simulink library "gbt_library"  (Simulink 7.4)
settings: Solver=ode45  StartTime=0.0  StopTime=10.0  RelTol=1e-3
libraries: xbsIndex_r4 x1525, casper_library_flow_control x20, casper_library_misc x15, xps_library x1
(part 4 of 14)

== system gbt_library/Parallel_CIC_filter_stage/comb_2 ==
  sync_in : Inport
  in1 : Inport  Port=2
  in2 : Inport  Port=3
  Delay2 : xbsIndex_r4/Delay  en=off  latency=1  dbl_ovrd=off  reg_retiming=off  block_type=delay
      settings: block_version=11.4
  sub_blk1 : xbsIndex_r4/AddSub  mode=Subtraction  use_carryin=off  use_carryout=off  en=off  latency=1  precision=User Defined  arith_type="Signed  (2's comp)"  n_bits=13  bin_pt=7  quantization=Truncate  overflow=Wrap  dbl_ovrd=off  use_behavioral_HDL=on  hw_selection=Fabric  pipelined=off  block_type=addsub
  sub_blk2 : xbsIndex_r4/AddSub  mode=Subtraction  use_carryin=off  use_carryout=off  en=off  latency=1  precision=User Defined  arith_type="Signed  (2's comp)"  n_bits=13  bin_pt=7  quantization=Truncate  overflow=Wrap  dbl_ovrd=off  use_behavioral_HDL=on  hw_selection=Fabric  pipelined=off  block_type=addsub
  sync_delay : xbsIndex_r4/Delay  en=off  latency=1  dbl_ovrd=off  reg_retiming=off  block_type=delay
      settings: block_version=11.4
  sync_out : Outport
  out1 : Outport  Port=2
  out2 : Outport  Port=3
  wires:
  in2/1 -> sub_blk2/1, Delay2/1
  in1/1 -> sub_blk2/2, sub_blk1/1
  sync_delay/1 -> sync_out/1
  sync_in/1 -> sync_delay/1
  sub_blk2/1 -> out2/1
  sub_blk1/1 -> out1/1
  Delay2/1 -> sub_blk1/2  "d_in2"

== system gbt_library/Parallel_CIC_filter_stage/comb_3 ==
  sync_in : Inport
  in1 : Inport  Port=2
  in2 : Inport  Port=3
  Delay2 : xbsIndex_r4/Delay  en=off  latency=1  dbl_ovrd=off  reg_retiming=off  block_type=delay
      settings: block_version=11.4
  sub_blk1 : xbsIndex_r4/AddSub  mode=Subtraction  use_carryin=off  use_carryout=off  en=off  latency=1  precision=User Defined  arith_type="Signed  (2's comp)"  n_bits=13  bin_pt=7  quantization=Truncate  overflow=Wrap  dbl_ovrd=off  use_behavioral_HDL=on  hw_selection=Fabric  pipelined=off  block_type=addsub
  sub_blk2 : xbsIndex_r4/AddSub  mode=Subtraction  use_carryin=off  use_carryout=off  en=off  latency=1  precision=User Defined  arith_type="Signed  (2's comp)"  n_bits=13  bin_pt=7  quantization=Truncate  overflow=Wrap  dbl_ovrd=off  use_behavioral_HDL=on  hw_selection=Fabric  pipelined=off  block_type=addsub
  sync_delay : xbsIndex_r4/Delay  en=off  latency=1  dbl_ovrd=off  reg_retiming=off  block_type=delay
      settings: block_version=11.4
  sync_out : Outport
  out1 : Outport  Port=2
  out2 : Outport  Port=3
  wires:
  in2/1 -> sub_blk2/1, Delay2/1
  in1/1 -> sub_blk2/2, sub_blk1/1
  sync_delay/1 -> sync_out/1
  sync_in/1 -> sync_delay/1
  sub_blk2/1 -> out2/1
  sub_blk1/1 -> out1/1
  Delay2/1 -> sub_blk1/2  "d_in2"

== system gbt_library/Parallel_CIC_filter_stage/downsample_3 ==
  sync_in : Inport
  In1 : Inport  Port=2
  In2 : Inport  Port=3
  Down_sample1 : xbsIndex_r4/Down Sample  sample_ratio=3  sample_phase="Last Value of Frame  (most efficient)"  en=off  latency=1  dbl_ovrd=off  block_type=dsamp
      settings: block_version=11.4
  Down_sample2 : xbsIndex_r4/Down Sample  sample_ratio=3  sample_phase="Last Value of Frame  (most efficient)"  en=off  latency=1  dbl_ovrd=off  block_type=dsamp
      settings: block_version=11.4
  delay1 : xbsIndex_r4/Delay  en=off  latency=1  dbl_ovrd=off  reg_retiming=off  block_type=delay
      settings: block_version=11.4
  delay2 : xbsIndex_r4/Delay  en=off  latency=0  dbl_ovrd=off  reg_retiming=off  block_type=delay
      settings: block_version=11.4
  sync_delay : xbsIndex_r4/Delay  en=off  latency=1  dbl_ovrd=off  reg_retiming=off  block_type=delay
      settings: block_version=11.4
  sync_out : Outport
  Out1 : Outport  Port=2
  Out2 : Outport  Port=3
  wires:
  sync_delay/1 -> sync_out/1
  sync_in/1 -> sync_delay/1
  Down_sample2/1 -> Out2/1
  delay2/1 -> Down_sample2/1  "dO2"
  In2/1 -> delay2/1
  Down_sample1/1 -> Out1/1
  delay1/1 -> Down_sample1/1  "dO1"
  In1/1 -> delay1/1

== system gbt_library/Parallel_CIC_filter_stage/int_1 ==
  in1 : Inport
  in2 : Inport  Port=2
  sync : Inport  Port=3
  Accumulator1 : xbsIndex_r4/Accumulator  operation=Add  n_bits=13  overflow=Wrap  scale=1  rst=off  hasbypass=off  en=off  dbl_ovrd=off  use_behavioral_HDL=on  implementation=Fabric  block_type=accum
      settings: block_version=11.4
  Accumulator2 : xbsIndex_r4/Accumulator  operation=Add  n_bits=13  overflow=Wrap  scale=1  rst=off  hasbypass=off  en=off  dbl_ovrd=off  use_behavioral_HDL=on  implementation=Fabric  block_type=accum
      settings: block_version=11.4
  Delay2 : xbsIndex_r4/Delay  en=off  latency=1  dbl_ovrd=off  reg_retiming=off  block_type=delay
      settings: block_version=11.4
  adder_tree1 : Subsystem
  adder_tree2 : Subsystem
  out1 : Outport
  out2 : Outport  Port=2
  wires:
  Accumulator2/1 -> adder_tree2/3(din_2), Delay2/1  "Im2"
  sync/1 -> adder_tree2/1(sync), adder_tree1/1(sync)
  Accumulator1/1 -> adder_tree2/2(din_1), adder_tree1/2(din_1)  "Im1"
  adder_tree2/2(dout) -> out2/1
  adder_tree1/2(dout) -> out1/1
  Delay2/1 -> adder_tree1/3(din_2)  "dIm2"
  in2/1 -> Accumulator2/1
  in1/1 -> Accumulator1/1

== system gbt_library/Parallel_CIC_filter_stage/int_2 ==
  in1 : Inport
  in2 : Inport  Port=2
  sync : Inport  Port=3
  Accumulator1 : xbsIndex_r4/Accumulator  operation=Add  n_bits=13  overflow=Wrap  scale=1  rst=off  hasbypass=off  en=off  dbl_ovrd=off  use_behavioral_HDL=on  implementation=Fabric  block_type=accum
      settings: block_version=11.4
  Accumulator2 : xbsIndex_r4/Accumulator  operation=Add  n_bits=13  overflow=Wrap  scale=1  rst=off  hasbypass=off  en=off  dbl_ovrd=off  use_behavioral_HDL=on  implementation=Fabric  block_type=accum
      settings: block_version=11.4
  Delay2 : xbsIndex_r4/Delay  en=off  latency=1  dbl_ovrd=off  reg_retiming=off  block_type=delay
      settings: block_version=11.4
  adder_tree1 : Subsystem
  adder_tree2 : Subsystem
  out1 : Outport
  out2 : Outport  Port=2
  wires:
  Accumulator2/1 -> adder_tree2/3(din_2), Delay2/1  "Im2"
  sync/1 -> adder_tree2/1(sync), adder_tree1/1(sync)
  Accumulator1/1 -> adder_tree2/2(din_1), adder_tree1/2(din_1)  "Im1"
  adder_tree2/2(dout) -> out2/1
  adder_tree1/2(dout) -> out1/1
  Delay2/1 -> adder_tree1/3(din_2)  "dIm2"
  in2/1 -> Accumulator2/1
  in1/1 -> Accumulator1/1

== system gbt_library/Parallel_CIC_filter_stage/int_3 ==
  in1 : Inport
  in2 : Inport  Port=2
  sync : Inport  Port=3
  Accumulator1 : xbsIndex_r4/Accumulator  operation=Add  n_bits=13  overflow=Wrap  scale=1  rst=off  hasbypass=off  en=off  dbl_ovrd=off  use_behavioral_HDL=on  implementation=Fabric  block_type=accum
      settings: block_version=11.4
  Accumulator2 : xbsIndex_r4/Accumulator  operation=Add  n_bits=13  overflow=Wrap  scale=1  rst=off  hasbypass=off  en=off  dbl_ovrd=off  use_behavioral_HDL=on  implementation=Fabric  block_type=accum
      settings: block_version=11.4
  Delay2 : xbsIndex_r4/Delay  en=off  latency=1  dbl_ovrd=off  reg_retiming=off  block_type=delay
      settings: block_version=11.4
  adder_tree1 : Subsystem
  adder_tree2 : Subsystem
  out1 : Outport
  out2 : Outport  Port=2
  wires:
  Accumulator2/1 -> adder_tree2/3(din_2), Delay2/1  "Im2"
  sync/1 -> adder_tree2/1(sync), adder_tree1/1(sync)
  Accumulator1/1 -> adder_tree2/2(din_1), adder_tree1/2(din_1)  "Im1"
  adder_tree2/2(dout) -> out2/1
  adder_tree1/2(dout) -> out1/1
  Delay2/1 -> adder_tree1/3(din_2)  "dIm2"
  in2/1 -> Accumulator2/1
  in1/1 -> Accumulator1/1

== system gbt_library/Spacketizer/parallel_to_serial_converter ==
  pin : Inport
  ld : Inport  Port=2
  shift : Inport  Port=3
  Logical : xbsIndex_r4/Logical  logical_function=OR  inputs=2  en=off  latency=0  precision=Full  arith_type=Unsigned  n_bits=16  bin_pt=0  align_bp=on  dbl_ovrd=off  block_type=logical
  filler : xbsIndex_r4/Constant  arith_type=Unsigned  const=0  n_bits=sout_width  bin_pt=0  explicit_period=on  period=1  equ=P=C  opselect=C  inp2=PCIN>>17  opr=+  inp1=P  carry=CIN  dbl_ovrd=off  block_type=constant
  shifter_unit1 : casper_library_flow_control/shifter_unit  SystemSampleTime=-1  data_width=64  pin_offset=0
  shifter_unit2 : casper_library_flow_control/shifter_unit  SystemSampleTime=-1  data_width=64  pin_offset=64
  shifter_unit3 : casper_library_flow_control/shifter_unit  SystemSampleTime=-1  data_width=64  pin_offset=128
  shifter_unit4 : casper_library_flow_control/shifter_unit  SystemSampleTime=-1  data_width=64  pin_offset=192
  sout : Outport  OutDataType=sfix(16)  OutScaling=2^0
  wires:
  shifter_unit4/1 -> sout/1
  shifter_unit3/1 -> shifter_unit4/2
  shifter_unit2/1 -> shifter_unit3/2
  shifter_unit1/1 -> shifter_unit2/2
  Logical/1 -> shifter_unit4/4, shifter_unit3/4, shifter_unit2/4, shifter_unit1/4
  pin/1 -> shifter_unit4/3, shifter_unit3/3, shifter_unit2/3, shifter_unit1/3
  filler/1 -> shifter_unit1/2
  shift/1 -> Logical/2
  ld/1 -> shifter_unit4/1, shifter_unit3/1, shifter_unit2/1, shifter_unit1/1, Logical/1

== system gbt_library/halfband/adder_tree ==
  sync : Inport
  din1 : Inport  Port=2
  din2 : Inport  Port=3
  din3 : Inport  Port=4
  din4 : Inport  Port=5
  addr1 : xbsIndex_r4/AddSub  mode=Addition  use_carryin=off  use_carryout=off  en=off  latency=1  precision=Full  arith_type=Unsigned  n_bits=16  bin_pt=14  quantization=Truncate  overflow=Wrap  dbl_ovrd=off  use_behavioral_HDL=off  hw_selection=Fabric  pipelined=on  use_rpm=on  block_type=addsub
  addr2 : xbsIndex_r4/AddSub  mode=Addition  use_carryin=off  use_carryout=off  en=off  latency=1  precision=Full  arith_type=Unsigned  n_bits=16  bin_pt=14  quantization=Truncate  overflow=Wrap  dbl_ovrd=off  use_behavioral_HDL=off  hw_selection=Fabric  pipelined=on  use_rpm=on  block_type=addsub
  addr3 : xbsIndex_r4/AddSub  mode=Addition  use_carryin=off  use_carryout=off  en=off  latency=1  precision=Full  arith_type=Unsigned  n_bits=16  bin_pt=14  quantization=Truncate  overflow=Wrap  dbl_ovrd=off  use_behavioral_HDL=off  hw_selection=Fabric  pipelined=on  use_rpm=on  block_type=addsub
  sync_delay : xbsIndex_r4/Delay  en=off  latency=2  dbl_ovrd=off  reg_retiming=on  block_type=delay
      settings: block_version=11.4
  sync_out : Outport
  dout : Outport  Port=2
  wires:
  addr3/1 -> dout/1  "adder_outs2_1"
  addr2/1 -> addr3/2  "adder_outs1_2"
  addr1/1 -> addr3/1  "adder_outs1_1"
  din4/1 -> addr2/2
  din3/1 -> addr2/1
  din2/1 -> addr1/2
  din1/1 -> addr1/1
  sync_delay/1 -> sync_out/1
  sync/1 -> sync_delay/1

== system gbt_library/halfband/adder_tree1 ==
  sync : Inport
  din1 : Inport  Port=2
  din2 : Inport  Port=3
  din3 : Inport  Port=4
  din4 : Inport  Port=5
  addr1 : xbsIndex_r4/AddSub  mode=Addition  use_carryin=off  use_carryout=off  en=off  latency=1  precision=Full  arith_type=Unsigned  n_bits=16  bin_pt=14  quantization=Truncate  overflow=Wrap  dbl_ovrd=off  use_behavioral_HDL=off  hw_selection=Fabric  pipelined=on  use_rpm=on  block_type=addsub
  addr2 : xbsIndex_r4/AddSub  mode=Addition  use_carryin=off  use_carryout=off  en=off  latency=1  precision=Full  arith_type=Unsigned  n_bits=16  bin_pt=14  quantization=Truncate  overflow=Wrap  dbl_ovrd=off  use_behavioral_HDL=off  hw_selection=Fabric  pipelined=on  use_rpm=on  block_type=addsub
  addr3 : xbsIndex_r4/AddSub  mode=Addition  use_carryin=off  use_carryout=off  en=off  latency=1  precision=Full  arith_type=Unsigned  n_bits=16  bin_pt=14  quantization=Truncate  overflow=Wrap  dbl_ovrd=off  use_behavioral_HDL=off  hw_selection=Fabric  pipelined=on  use_rpm=on  block_type=addsub
  sync_delay : xbsIndex_r4/Delay  en=off  latency=2  dbl_ovrd=off  reg_retiming=on  block_type=delay
      settings: block_version=11.4
  sync_out : Outport
  dout : Outport  Port=2
  wires:
  addr3/1 -> dout/1  "adder_outs2_1"
  addr2/1 -> addr3/2  "adder_outs1_2"
  addr1/1 -> addr3/1  "adder_outs1_1"
  din4/1 -> addr2/2
  din3/1 -> addr2/1
  din2/1 -> addr1/2
  din1/1 -> addr1/1
  sync_delay/1 -> sync_out/1
  sync/1 -> sync_delay/1

== system gbt_library/halfband/adder_tree3 ==
  sync : Inport
  din1 : Inport  Port=2
  din2 : Inport  Port=3
  din3 : Inport  Port=4
  din4 : Inport  Port=5
  addr1 : xbsIndex_r4/AddSub  mode=Addition  use_carryin=off  use_carryout=off  en=off  latency=1  precision=Full  arith_type=Unsigned  n_bits=16  bin_pt=14  quantization=Truncate  overflow=Wrap  dbl_ovrd=off  use_behavioral_HDL=off  hw_selection=Fabric  pipelined=on  use_rpm=on  block_type=addsub
  addr2 : xbsIndex_r4/AddSub  mode=Addition  use_carryin=off  use_carryout=off  en=off  latency=1  precision=Full  arith_type=Unsigned  n_bits=16  bin_pt=14  quantization=Truncate  overflow=Wrap  dbl_ovrd=off  use_behavioral_HDL=off  hw_selection=Fabric  pipelined=on  use_rpm=on  block_type=addsub
  addr3 : xbsIndex_r4/AddSub  mode=Addition  use_carryin=off  use_carryout=off  en=off  latency=1  precision=Full  arith_type=Unsigned  n_bits=16  bin_pt=14  quantization=Truncate  overflow=Wrap  dbl_ovrd=off  use_behavioral_HDL=off  hw_selection=Fabric  pipelined=on  use_rpm=on  block_type=addsub
  sync_delay : xbsIndex_r4/Delay  en=off  latency=2  dbl_ovrd=off  reg_retiming=on  block_type=delay
      settings: block_version=11.4
  sync_out : Outport
  dout : Outport  Port=2
  wires:
  addr3/1 -> dout/1  "adder_outs2_1"
  addr2/1 -> addr3/2  "adder_outs1_2"
  addr1/1 -> addr3/1  "adder_outs1_1"
  din4/1 -> addr2/2
  din3/1 -> addr2/1
  din2/1 -> addr1/2
  din1/1 -> addr1/1
  sync_delay/1 -> sync_out/1
  sync/1 -> sync_delay/1

== system gbt_library/halfband/adder_tree4 ==
  sync : Inport
  din1 : Inport  Port=2
  din2 : Inport  Port=3
  din3 : Inport  Port=4
  din4 : Inport  Port=5
  addr1 : xbsIndex_r4/AddSub  mode=Addition  use_carryin=off  use_carryout=off  en=off  latency=1  precision=Full  arith_type=Unsigned  n_bits=16  bin_pt=14  quantization=Truncate  overflow=Wrap  dbl_ovrd=off  use_behavioral_HDL=off  hw_selection=Fabric  pipelined=on  use_rpm=on  block_type=addsub
  addr2 : xbsIndex_r4/AddSub  mode=Addition  use_carryin=off  use_carryout=off  en=off  latency=1  precision=Full  arith_type=Unsigned  n_bits=16  bin_pt=14  quantization=Truncate  overflow=Wrap  dbl_ovrd=off  use_behavioral_HDL=off  hw_selection=Fabric  pipelined=on  use_rpm=on  block_type=addsub
  addr3 : xbsIndex_r4/AddSub  mode=Addition  use_carryin=off  use_carryout=off  en=off  latency=1  precision=Full  arith_type=Unsigned  n_bits=16  bin_pt=14  quantization=Truncate  overflow=Wrap  dbl_ovrd=off  use_behavioral_HDL=off  hw_selection=Fabric  pipelined=on  use_rpm=on  block_type=addsub
  sync_delay : xbsIndex_r4/Delay  en=off  latency=2  dbl_ovrd=off  reg_retiming=on  block_type=delay
      settings: block_version=11.4
  sync_out : Outport
  dout : Outport  Port=2
  wires:
  addr3/1 -> dout/1  "adder_outs2_1"
  addr2/1 -> addr3/2  "adder_outs1_2"
  addr1/1 -> addr3/1  "adder_outs1_1"
  din4/1 -> addr2/2
  din3/1 -> addr2/1
  din2/1 -> addr1/2
  din1/1 -> addr1/1
  sync_delay/1 -> sync_out/1
  sync/1 -> sync_delay/1

== system gbt_library/halfband/parallel_fir ==
  sync_in : Inport
  in1 : Inport  Port=2
  in2 : Inport  Port=3
  AddSub{1,3,5..6} (4 alike) : xbsIndex_r4/AddSub  mode=Subtraction  use_carryin=off  use_carryout=off  en=off  latency=0  precision=Full  arith_type=Unsigned  n_bits=16  bin_pt=14  quantization=Truncate  overflow=Wrap  dbl_ovrd=off  use_behavioral_HDL=off  hw_selection=Fabric  pipelined=off  block_type=addsub
  AddSub2 : xbsIndex_r4/AddSub  mode=Addition  use_carryin=off  use_carryout=off  en=off  latency=0  precision=Full  arith_type=Unsigned  n_bits=16  bin_pt=14  quantization=Truncate  overflow=Wrap  dbl_ovrd=off  use_behavioral_HDL=off  hw_selection=Fabric  pipelined=off  block_type=addsub
  AddSub4 : xbsIndex_r4/AddSub  mode=Addition  use_carryin=off  use_carryout=off  en=off  latency=0  precision=Full  arith_type=Unsigned  n_bits=16  bin_pt=14  quantization=Truncate  overflow=Wrap  dbl_ovrd=off  use_behavioral_HDL=off  hw_selection=Fabric  pipelined=off  block_type=addsub
  Add_imag_in12 : xbsIndex_r4/AddSub  mode=Addition  use_carryin=off  use_carryout=off  en=off  latency=0  precision=Full  arith_type=Unsigned  n_bits=16  bin_pt=14  quantization=Truncate  overflow=Wrap  dbl_ovrd=off  use_behavioral_HDL=off  hw_selection=Fabric  pipelined=off  block_type=addsub
  Add_real_in12 : xbsIndex_r4/AddSub  mode=Addition  use_carryin=off  use_carryout=off  en=off  latency=0  precision=Full  arith_type=Unsigned  n_bits=16  bin_pt=14  quantization=Truncate  overflow=Wrap  dbl_ovrd=off  use_behavioral_HDL=off  hw_selection=Fabric  pipelined=off  block_type=addsub
  Delay : xbsIndex_r4/Delay  en=off  latency=1  dbl_ovrd=off  reg_retiming=off  block_type=delay
      settings: block_version=11.4
  Delay1 : xbsIndex_r4/Delay  en=off  latency=1  dbl_ovrd=off  reg_retiming=off  block_type=delay
      settings: block_version=11.4
  c_to_ri : Subsystem
  c_to_ri1 : Subsystem
  c_to_ri_f0 : Subsystem
  c_to_ri_f0pf1 : Subsystem
  c_to_ri_f1 : Subsystem
  f0 : Subsystem
      settings: AttributesFormatString=|
      | 2 taps
      | 4_3 r/i
  f0pf1 : Subsystem
      settings: AttributesFormatString=|
      | 2 taps
      | 4_3 r/i
  f1 : Subsystem
      settings: AttributesFormatString=|
      | 2 taps
      | 4_3 r/i
  sync_out : Outport
  y0r : Outport  Port=2
  y0i : Outport  Port=3
  y1r : Outport  Port=4
  y1i : Outport  Port=5
  wires:
  c_to_ri/1(re) -> f0/2(real1), Add_real_in12/1  "real_in1"
  c_to_ri1/1(re) -> f1/2(real1), Add_real_in12/2  "real_in2"
  c_to_ri/2(im) -> f0/3(imag1), Add_imag_in12/1  "imag_in1"
  c_to_ri1/2(im) -> f1/3(imag1), Add_imag_in12/2  "imag_in2"
  sync_in/1 -> f1/1(sync_in), f0pf1/1(sync_in), f0/1(sync_in)
  c_to_ri_f1/1(re) -> AddSub1/2, Delay/1  "real_f1_out"
  c_to_ri_f1/2(im) -> AddSub3/2, Delay1/1  "imag_f1_out"
  c_to_ri_f0/1(re) -> AddSub5/1, AddSub2/1  "real_f0_out"
  c_to_ri_f0/2(im) -> AddSub6/1, AddSub4/1  "imag_f0_out"
  AddSub6/1 -> y1i/1
  AddSub3/1 -> AddSub6/2
  AddSub5/1 -> y1r/1
  AddSub1/1 -> AddSub5/2
  AddSub4/1 -> y0i/1
  Delay1/1 -> AddSub4/2  "imag_f1_out_delayed"
  c_to_ri_f0pf1/2(im) -> AddSub3/1  "imag_f0pf1_out"
  AddSub2/1 -> y0r/1
  Delay/1 -> AddSub2/2  "real_f1_out_delayed"
  c_to_ri_f0pf1/1(re) -> AddSub1/1  "real_f0pf1_out"
  f0pf1/2(dout) -> c_to_ri_f0pf1/1(c)  "f0pf1_out"
  f0/2(dout) -> c_to_ri_f0/1(c)  "f0_out"
  f1/2(dout) -> c_to_ri_f1/1(c)  "f1_out"
  Add_imag_in12/1 -> f0pf1/3(imag1)  "imag_in12"
  Add_real_in12/1 -> f0pf1/2(real1)  "real_in12"
  f0/1(sync_out) -> sync_out/1
  in2/1 -> c_to_ri1/1(c)
  in1/1 -> c_to_ri/1(c)

== system gbt_library/halfband/parallel_fir1 ==
  sync_in : Inport
  in1 : Inport  Port=2
  in2 : Inport  Port=3
  AddSub{1,3,5..6} (4 alike) : xbsIndex_r4/AddSub  mode=Subtraction  use_carryin=off  use_carryout=off  en=off  latency=0  precision=Full  arith_type=Unsigned  n_bits=16  bin_pt=14  quantization=Truncate  overflow=Wrap  dbl_ovrd=off  use_behavioral_HDL=off  hw_selection=Fabric  pipelined=off  block_type=addsub
  AddSub2 : xbsIndex_r4/AddSub  mode=Addition  use_carryin=off  use_carryout=off  en=off  latency=0  precision=Full  arith_type=Unsigned  n_bits=16  bin_pt=14  quantization=Truncate  overflow=Wrap  dbl_ovrd=off  use_behavioral_HDL=off  hw_selection=Fabric  pipelined=off  block_type=addsub
  AddSub4 : xbsIndex_r4/AddSub  mode=Addition  use_carryin=off  use_carryout=off  en=off  latency=0  precision=Full  arith_type=Unsigned  n_bits=16  bin_pt=14  quantization=Truncate  overflow=Wrap  dbl_ovrd=off  use_behavioral_HDL=off  hw_selection=Fabric  pipelined=off  block_type=addsub
  Add_imag_in12 : xbsIndex_r4/AddSub  mode=Addition  use_carryin=off  use_carryout=off  en=off  latency=0  precision=Full  arith_type=Unsigned  n_bits=16  bin_pt=14  quantization=Truncate  overflow=Wrap  dbl_ovrd=off  use_behavioral_HDL=off  hw_selection=Fabric  pipelined=off  block_type=addsub
  Add_real_in12 : xbsIndex_r4/AddSub  mode=Addition  use_carryin=off  use_carryout=off  en=off  latency=0  precision=Full  arith_type=Unsigned  n_bits=16  bin_pt=14  quantization=Truncate  overflow=Wrap  dbl_ovrd=off  use_behavioral_HDL=off  hw_selection=Fabric  pipelined=off  block_type=addsub
  Delay : xbsIndex_r4/Delay  en=off  latency=1  dbl_ovrd=off  reg_retiming=off  block_type=delay
      settings: block_version=11.4
  Delay1 : xbsIndex_r4/Delay  en=off  latency=1  dbl_ovrd=off  reg_retiming=off  block_type=delay
      settings: block_version=11.4
  c_to_ri : Subsystem
  c_to_ri1 : Subsystem
  c_to_ri_f0 : Subsystem
  c_to_ri_f0pf1 : Subsystem
  c_to_ri_f1 : Subsystem
  f0 : Subsystem
      settings: AttributesFormatString=|
      | 2 taps
      | 4_3 r/i
  f0pf1 : Subsystem
      settings: AttributesFormatString=|
      | 2 taps
      | 4_3 r/i
  f1 : Subsystem
      settings: AttributesFormatString=|
      | 2 taps
      | 4_3 r/i
  sync_out : Outport
  y0r : Outport  Port=2
  y0i : Outport  Port=3
  y1r : Outport  Port=4
  y1i : Outport  Port=5
  wires:
  c_to_ri/1(re) -> f0/2(real1), Add_real_in12/1  "real_in1"
  c_to_ri1/1(re) -> f1/2(real1), Add_real_in12/2  "real_in2"
  c_to_ri/2(im) -> f0/3(imag1), Add_imag_in12/1  "imag_in1"
  c_to_ri1/2(im) -> f1/3(imag1), Add_imag_in12/2  "imag_in2"
  sync_in/1 -> f1/1(sync_in), f0pf1/1(sync_in), f0/1(sync_in)
  c_to_ri_f1/1(re) -> AddSub1/2, Delay/1  "real_f1_out"
  c_to_ri_f1/2(im) -> AddSub3/2, Delay1/1  "imag_f1_out"
  c_to_ri_f0/1(re) -> AddSub5/1, AddSub2/1  "real_f0_out"
  c_to_ri_f0/2(im) -> AddSub6/1, AddSub4/1  "imag_f0_out"
  AddSub6/1 -> y1i/1
  AddSub3/1 -> AddSub6/2
  AddSub5/1 -> y1r/1
  AddSub1/1 -> AddSub5/2
  AddSub4/1 -> y0i/1
  Delay1/1 -> AddSub4/2  "imag_f1_out_delayed"
  c_to_ri_f0pf1/2(im) -> AddSub3/1  "imag_f0pf1_out"
  AddSub2/1 -> y0r/1
  Delay/1 -> AddSub2/2  "real_f1_out_delayed"
  c_to_ri_f0pf1/1(re) -> AddSub1/1  "real_f0pf1_out"
  f0pf1/2(dout) -> c_to_ri_f0pf1/1(c)  "f0pf1_out"
  f0/2(dout) -> c_to_ri_f0/1(c)  "f0_out"
  f1/2(dout) -> c_to_ri_f1/1(c)  "f1_out"
  Add_imag_in12/1 -> f0pf1/3(imag1)  "imag_in12"
  Add_real_in12/1 -> f0pf1/2(real1)  "real_in12"
  f0/1(sync_out) -> sync_out/1
  in2/1 -> c_to_ri1/1(c)
  in1/1 -> c_to_ri/1(c)

== system gbt_library/halfband/parallel_fir2 ==
  sync_in : Inport
  in1 : Inport  Port=2
  in2 : Inport  Port=3
  AddSub{1,3,5..6} (4 alike) : xbsIndex_r4/AddSub  mode=Subtraction  use_carryin=off  use_carryout=off  en=off  latency=0  precision=Full  arith_type=Unsigned  n_bits=16  bin_pt=14  quantization=Truncate  overflow=Wrap  dbl_ovrd=off  use_behavioral_HDL=off  hw_selection=Fabric  pipelined=off  block_type=addsub
  AddSub2 : xbsIndex_r4/AddSub  mode=Addition  use_carryin=off  use_carryout=off  en=off  latency=0  precision=Full  arith_type=Unsigned  n_bits=16  bin_pt=14  quantization=Truncate  overflow=Wrap  dbl_ovrd=off  use_behavioral_HDL=off  hw_selection=Fabric  pipelined=off  block_type=addsub
  AddSub4 : xbsIndex_r4/AddSub  mode=Addition  use_carryin=off  use_carryout=off  en=off  latency=0  precision=Full  arith_type=Unsigned  n_bits=16  bin_pt=14  quantization=Truncate  overflow=Wrap  dbl_ovrd=off  use_behavioral_HDL=off  hw_selection=Fabric  pipelined=off  block_type=addsub
  Add_imag_in12 : xbsIndex_r4/AddSub  mode=Addition  use_carryin=off  use_carryout=off  en=off  latency=0  precision=Full  arith_type=Unsigned  n_bits=16  bin_pt=14  quantization=Truncate  overflow=Wrap  dbl_ovrd=off  use_behavioral_HDL=off  hw_selection=Fabric  pipelined=off  block_type=addsub
  Add_real_in12 : xbsIndex_r4/AddSub  mode=Addition  use_carryin=off  use_carryout=off  en=off  latency=0  precision=Full  arith_type=Unsigned  n_bits=16  bin_pt=14  quantization=Truncate  overflow=Wrap  dbl_ovrd=off  use_behavioral_HDL=off  hw_selection=Fabric  pipelined=off  block_type=addsub
  Delay : xbsIndex_r4/Delay  en=off  latency=1  dbl_ovrd=off  reg_retiming=off  block_type=delay
      settings: block_version=11.4
  Delay1 : xbsIndex_r4/Delay  en=off  latency=1  dbl_ovrd=off  reg_retiming=off  block_type=delay
      settings: block_version=11.4
  c_to_ri : Subsystem
  c_to_ri1 : Subsystem
  c_to_ri_f0 : Subsystem
  c_to_ri_f0pf1 : Subsystem
  c_to_ri_f1 : Subsystem
  f0 : Subsystem
      settings: AttributesFormatString=|
      | 2 taps
      | 4_3 r/i
  f0pf1 : Subsystem
      settings: AttributesFormatString=|
      | 2 taps
      | 4_3 r/i
  f1 : Subsystem
      settings: AttributesFormatString=|
      | 2 taps
      | 4_3 r/i
  sync_out : Outport
  y0r : Outport  Port=2
  y0i : Outport  Port=3
  y1r : Outport  Port=4
  y1i : Outport  Port=5
  wires:
  c_to_ri/1(re) -> f0/2(real1), Add_real_in12/1  "real_in1"
  c_to_ri1/1(re) -> f1/2(real1), Add_real_in12/2  "real_in2"
  c_to_ri/2(im) -> f0/3(imag1), Add_imag_in12/1  "imag_in1"
  c_to_ri1/2(im) -> f1/3(imag1), Add_imag_in12/2  "imag_in2"
  sync_in/1 -> f1/1(sync_in), f0pf1/1(sync_in), f0/1(sync_in)
  c_to_ri_f1/1(re) -> AddSub1/2, Delay/1  "real_f1_out"
  c_to_ri_f1/2(im) -> AddSub3/2, Delay1/1  "imag_f1_out"
  c_to_ri_f0/1(re) -> AddSub5/1, AddSub2/1  "real_f0_out"
  c_to_ri_f0/2(im) -> AddSub6/1, AddSub4/1  "imag_f0_out"
  AddSub6/1 -> y1i/1
  AddSub3/1 -> AddSub6/2
  AddSub5/1 -> y1r/1
  AddSub1/1 -> AddSub5/2
  AddSub4/1 -> y0i/1
  Delay1/1 -> AddSub4/2  "imag_f1_out_delayed"
  c_to_ri_f0pf1/2(im) -> AddSub3/1  "imag_f0pf1_out"
  AddSub2/1 -> y0r/1
  Delay/1 -> AddSub2/2  "real_f1_out_delayed"
  c_to_ri_f0pf1/1(re) -> AddSub1/1  "real_f0pf1_out"
  f0pf1/2(dout) -> c_to_ri_f0pf1/1(c)  "f0pf1_out"
  f0/2(dout) -> c_to_ri_f0/1(c)  "f0_out"
  f1/2(dout) -> c_to_ri_f1/1(c)  "f1_out"
  Add_imag_in12/1 -> f0pf1/3(imag1)  "imag_in12"
  Add_real_in12/1 -> f0pf1/2(real1)  "real_in12"
  f0/1(sync_out) -> sync_out/1
  in2/1 -> c_to_ri1/1(c)
  in1/1 -> c_to_ri/1(c)

== system gbt_library/halfband/parallel_fir3 ==
  sync_in : Inport
  in1 : Inport  Port=2
  in2 : Inport  Port=3
  AddSub{1,3,5..6} (4 alike) : xbsIndex_r4/AddSub  mode=Subtraction  use_carryin=off  use_carryout=off  en=off  latency=0  precision=Full  arith_type=Unsigned  n_bits=16  bin_pt=14  quantization=Truncate  overflow=Wrap  dbl_ovrd=off  use_behavioral_HDL=off  hw_selection=Fabric  pipelined=off  block_type=addsub
  AddSub2 : xbsIndex_r4/AddSub  mode=Addition  use_carryin=off  use_carryout=off  en=off  latency=0  precision=Full  arith_type=Unsigned  n_bits=16  bin_pt=14  quantization=Truncate  overflow=Wrap  dbl_ovrd=off  use_behavioral_HDL=off  hw_selection=Fabric  pipelined=off  block_type=addsub
  AddSub4 : xbsIndex_r4/AddSub  mode=Addition  use_carryin=off  use_carryout=off  en=off  latency=0  precision=Full  arith_type=Unsigned  n_bits=16  bin_pt=14  quantization=Truncate  overflow=Wrap  dbl_ovrd=off  use_behavioral_HDL=off  hw_selection=Fabric  pipelined=off  block_type=addsub
  Add_imag_in12 : xbsIndex_r4/AddSub  mode=Addition  use_carryin=off  use_carryout=off  en=off  latency=0  precision=Full  arith_type=Unsigned  n_bits=16  bin_pt=14  quantization=Truncate  overflow=Wrap  dbl_ovrd=off  use_behavioral_HDL=off  hw_selection=Fabric  pipelined=off  block_type=addsub
  Add_real_in12 : xbsIndex_r4/AddSub  mode=Addition  use_carryin=off  use_carryout=off  en=off  latency=0  precision=Full  arith_type=Unsigned  n_bits=16  bin_pt=14  quantization=Truncate  overflow=Wrap  dbl_ovrd=off  use_behavioral_HDL=off  hw_selection=Fabric  pipelined=off  block_type=addsub
  Delay : xbsIndex_r4/Delay  en=off  latency=1  dbl_ovrd=off  reg_retiming=off  block_type=delay
      settings: block_version=11.4
  Delay1 : xbsIndex_r4/Delay  en=off  latency=1  dbl_ovrd=off  reg_retiming=off  block_type=delay
      settings: block_version=11.4
  c_to_ri : Subsystem
  c_to_ri1 : Subsystem
  c_to_ri_f0 : Subsystem
  c_to_ri_f0pf1 : Subsystem
  c_to_ri_f1 : Subsystem
  f0 : Subsystem
      settings: AttributesFormatString=|
      | 2 taps
      | 4_3 r/i
  f0pf1 : Subsystem
      settings: AttributesFormatString=|
      | 2 taps
      | 4_3 r/i
  f1 : Subsystem
      settings: AttributesFormatString=|
      | 2 taps
      | 4_3 r/i
  sync_out : Outport
  y0r : Outport  Port=2
  y0i : Outport  Port=3
  y1r : Outport  Port=4
  y1i : Outport  Port=5
  wires:
  c_to_ri/1(re) -> f0/2(real1), Add_real_in12/1  "real_in1"
  c_to_ri1/1(re) -> f1/2(real1), Add_real_in12/2  "real_in2"
  c_to_ri/2(im) -> f0/3(imag1), Add_imag_in12/1  "imag_in1"
  c_to_ri1/2(im) -> f1/3(imag1), Add_imag_in12/2  "imag_in2"
  sync_in/1 -> f1/1(sync_in), f0pf1/1(sync_in), f0/1(sync_in)
  c_to_ri_f1/1(re) -> AddSub1/2, Delay/1  "real_f1_out"
  c_to_ri_f1/2(im) -> AddSub3/2, Delay1/1  "imag_f1_out"
  c_to_ri_f0/1(re) -> AddSub5/1, AddSub2/1  "real_f0_out"
  c_to_ri_f0/2(im) -> AddSub6/1, AddSub4/1  "imag_f0_out"
  AddSub6/1 -> y1i/1
  AddSub3/1 -> AddSub6/2
  AddSub5/1 -> y1r/1
  AddSub1/1 -> AddSub5/2
  AddSub4/1 -> y0i/1
  Delay1/1 -> AddSub4/2  "imag_f1_out_delayed"
  c_to_ri_f0pf1/2(im) -> AddSub3/1  "imag_f0pf1_out"
  AddSub2/1 -> y0r/1
  Delay/1 -> AddSub2/2  "real_f1_out_delayed"
  c_to_ri_f0pf1/1(re) -> AddSub1/1  "real_f0pf1_out"
  f0pf1/2(dout) -> c_to_ri_f0pf1/1(c)  "f0pf1_out"
  f0/2(dout) -> c_to_ri_f0/1(c)  "f0_out"
  f1/2(dout) -> c_to_ri_f1/1(c)  "f1_out"
  Add_imag_in12/1 -> f0pf1/3(imag1)  "imag_in12"
  Add_real_in12/1 -> f0pf1/2(real1)  "real_in12"
  f0/1(sync_out) -> sync_out/1
  in2/1 -> c_to_ri1/1(c)
  in1/1 -> c_to_ri/1(c)

== system gbt_library/parallel_fir/c_to_ri ==
  c : Inport
  force_im : xbsIndex_r4/Reinterpret  force_arith_type=on  arith_type="Signed  (2's comp)"  force_bin_pt=on  bin_pt=7  block_type=reinterpret
      settings: infoedit="Changes signal type without altering the binary representation.   You can changed the signal between signed and unsigned, and relocate the binary point.<br><br>Hardware notes: In hardware this block costs nothing.<br><br>Example:  Suppose the input is 6 bits wide, signed, with 2 fractional bits, and the output is forced to unsigned with 0 fractional bits.  Then an input of -2.0 (1110.00 in binary 2's complement) becomes an output of 56 (111000 in binary)."
  force_re : xbsIndex_r4/Reinterpret  force_arith_type=on  arith_type="Signed  (2's comp)"  force_bin_pt=on  bin_pt=7  block_type=reinterpret
      settings: infoedit="Changes signal type without altering the binary representation.   You can changed the signal between signed and unsigned, and relocate the binary point.<br><br>Hardware notes: In hardware this block costs nothing.<br><br>Example:  Suppose the input is 6 bits wide, signed, with 2 fractional bits, and the output is forced to unsigned with 0 fractional bits.  Then an input of -2.0 (1110.00 in binary 2's complement) becomes an output of 56 (111000 in binary)."
  slice_im : xbsIndex_r4/Slice  nbits=8  boolean_output=off  mode=Lower Bit Location + Width  bit1=0  base1=MSB of Input  bit0=0  base0=LSB of Input  dbl_ovrd=off  block_type=slice
  slice_re : xbsIndex_r4/Slice  nbits=8  boolean_output=off  mode=Upper Bit Location + Width  bit1=0  base1=MSB of Input  bit0=0  base0=LSB of Input  dbl_ovrd=off  block_type=slice
  re : Outport
  im : Outport  Port=2
  wires:
  c/1 -> slice_re/1, slice_im/1
  slice_re/1 -> force_re/1
  slice_im/1 -> force_im/1
  force_re/1 -> re/1
  force_im/1 -> im/1

== system gbt_library/parallel_fir/c_to_ri1 ==
  c : Inport
  force_im : xbsIndex_r4/Reinterpret  force_arith_type=on  arith_type="Signed  (2's comp)"  force_bin_pt=on  bin_pt=7  block_type=reinterpret
      settings: infoedit="Changes signal type without altering the binary representation.   You can changed the signal between signed and unsigned, and relocate the binary point.<br><br>Hardware notes: In hardware this block costs nothing.<br><br>Example:  Suppose the input is 6 bits wide, signed, with 2 fractional bits, and the output is forced to unsigned with 0 fractional bits.  Then an input of -2.0 (1110.00 in binary 2's complement) becomes an output of 56 (111000 in binary)."
  force_re : xbsIndex_r4/Reinterpret  force_arith_type=on  arith_type="Signed  (2's comp)"  force_bin_pt=on  bin_pt=7  block_type=reinterpret
      settings: infoedit="Changes signal type without altering the binary representation.   You can changed the signal between signed and unsigned, and relocate the binary point.<br><br>Hardware notes: In hardware this block costs nothing.<br><br>Example:  Suppose the input is 6 bits wide, signed, with 2 fractional bits, and the output is forced to unsigned with 0 fractional bits.  Then an input of -2.0 (1110.00 in binary 2's complement) becomes an output of 56 (111000 in binary)."
  slice_im : xbsIndex_r4/Slice  nbits=8  boolean_output=off  mode=Lower Bit Location + Width  bit1=0  base1=MSB of Input  bit0=0  base0=LSB of Input  dbl_ovrd=off  block_type=slice
  slice_re : xbsIndex_r4/Slice  nbits=8  boolean_output=off  mode=Upper Bit Location + Width  bit1=0  base1=MSB of Input  bit0=0  base0=LSB of Input  dbl_ovrd=off  block_type=slice
  re : Outport
  im : Outport  Port=2
  wires:
  c/1 -> slice_re/1, slice_im/1
  slice_re/1 -> force_re/1
  slice_im/1 -> force_im/1
  force_re/1 -> re/1
  force_im/1 -> im/1

== system gbt_library/parallel_fir/c_to_ri2 ==
  c : Inport
  force_im : xbsIndex_r4/Reinterpret  force_arith_type=on  arith_type="Signed  (2's comp)"  force_bin_pt=on  bin_pt=7  block_type=reinterpret
      settings: infoedit="Changes signal type without altering the binary representation.   You can changed the signal between signed and unsigned, and relocate the binary point.<br><br>Hardware notes: In hardware this block costs nothing.<br><br>Example:  Suppose the input is 6 bits wide, signed, with 2 fractional bits, and the output is forced to unsigned with 0 fractional bits.  Then an input of -2.0 (1110.00 in binary 2's complement) becomes an output of 56 (111000 in binary)."
  force_re : xbsIndex_r4/Reinterpret  force_arith_type=on  arith_type="Signed  (2's comp)"  force_bin_pt=on  bin_pt=7  block_type=reinterpret
      settings: infoedit="Changes signal type without altering the binary representation.   You can changed the signal between signed and unsigned, and relocate the binary point.<br><br>Hardware notes: In hardware this block costs nothing.<br><br>Example:  Suppose the input is 6 bits wide, signed, with 2 fractional bits, and the output is forced to unsigned with 0 fractional bits.  Then an input of -2.0 (1110.00 in binary 2's complement) becomes an output of 56 (111000 in binary)."
  slice_im : xbsIndex_r4/Slice  nbits=8  boolean_output=off  mode=Lower Bit Location + Width  bit1=0  base1=MSB of Input  bit0=0  base0=LSB of Input  dbl_ovrd=off  block_type=slice
  slice_re : xbsIndex_r4/Slice  nbits=8  boolean_output=off  mode=Upper Bit Location + Width  bit1=0  base1=MSB of Input  bit0=0  base0=LSB of Input  dbl_ovrd=off  block_type=slice
  re : Outport
  im : Outport  Port=2
  wires:
  c/1 -> slice_re/1, slice_im/1
  slice_re/1 -> force_re/1
  slice_im/1 -> force_im/1
  force_re/1 -> re/1
  force_im/1 -> im/1

== system gbt_library/parallel_fir/f0 ==
  sync_in : Inport
  real1 : Inport  Port=2
  imag1 : Inport  Port=3
  convert1 : xbsIndex_r4/Convert  arith_type="Signed  (2's comp)"  n_bits=4  bin_pt=3  quantization=Truncate  overflow=Wrap  latency=1  dbl_ovrd=off  pipeline=off  block_type=convert
      settings: block_version=11.4
  convert2 : xbsIndex_r4/Convert  arith_type="Signed  (2's comp)"  n_bits=4  bin_pt=3  quantization=Truncate  overflow=Wrap  latency=1  dbl_ovrd=off  pipeline=off  block_type=convert
      settings: block_version=11.4
  delay : xbsIndex_r4/Delay  en=off  latency=3  dbl_ovrd=off  reg_retiming=off  block_type=delay
      settings: block_version=11.4
  fir_col1 : Subsystem
  fir_col2 : Subsystem
  fir_col3 : Subsystem
  fir_col4 : Subsystem
  imag_sum : Subsystem
      settings: AttributesFormatString=latency 2
  real_sum : Subsystem
      settings: AttributesFormatString=latency 2
  ri_to_c : Subsystem
  shift1 : xbsIndex_r4/Shift  shift_dir=Left  shift_bits=1  en=off  latency=0  precision=Full  arith_type="Signed  (2's comp)"  n_bits=16  bin_pt=14  quantization=Truncate  overflow=Wrap  dbl_ovrd=off  block_type=shift
  shift2 : xbsIndex_r4/Shift  shift_dir=Left  shift_bits=1  en=off  latency=0  precision=Full  arith_type="Signed  (2's comp)"  n_bits=16  bin_pt=14  quantization=Truncate  overflow=Wrap  dbl_ovrd=off  block_type=shift
  sync_out : Outport
  dout : Outport  Port=2
  wires:
  delay/1 -> real_sum/1(sync), imag_sum/1(sync)
  shift2/1 -> convert2/1
  imag_sum/2(dout) -> shift2/1
  shift1/1 -> convert1/1
  real_sum/2(dout) -> shift1/1
  ri_to_c/1(c) -> dout/1
  convert2/1 -> ri_to_c/2(im)
  convert1/1 -> ri_to_c/1(re)
  real_sum/1(sync_out) -> sync_out/1
  fir_col4/3(real_sum) -> real_sum/5(din4)  "xlsub2_real_sum_inports5"
  fir_col3/3(real_sum) -> real_sum/4(din3)  "xlsub2_real_sum_inports4"
  fir_col2/3(real_sum) -> real_sum/3(din2)  "xlsub2_real_sum_inports3"
  fir_col1/3(real_sum) -> real_sum/2(din1)  "xlsub2_real_sum_inports2"
  fir_col4/4(imag_sum) -> imag_sum/5(din4)  "xlsub2_imag_sum_inports5"
  fir_col3/4(imag_sum) -> imag_sum/4(din3)  "xlsub2_imag_sum_inports4"
  fir_col2/4(imag_sum) -> imag_sum/3(din2)  "xlsub2_imag_sum_inports3"
  fir_col1/4(imag_sum) -> imag_sum/2(din1)  "xlsub2_imag_sum_inports2"
  fir_col3/2(imag_out1) -> fir_col4/2(imag1)  "xlsub2_fir_col3_2"
  fir_col3/1(real_out1) -> fir_col4/1(real1)  "xlsub2_fir_col3_1"
  fir_col2/2(imag_out1) -> fir_col3/2(imag1)  "xlsub2_fir_col2_2"
  fir_col2/1(real_out1) -> fir_col3/1(real1)  "xlsub2_fir_col2_1"
  fir_col1/2(imag_out1) -> fir_col2/2(imag1)  "xlsub2_fir_col1_2"
  fir_col1/1(real_out1) -> fir_col2/1(real1)  "xlsub2_fir_col1_1"
  imag1/1 -> fir_col1/2(imag1)
  real1/1 -> fir_col1/1(real1)
  sync_in/1 -> delay/1

== system gbt_library/parallel_fir/f0pf1 ==
  sync_in : Inport
  real1 : Inport  Port=2
  imag1 : Inport  Port=3
  convert1 : xbsIndex_r4/Convert  arith_type="Signed  (2's comp)"  n_bits=4  bin_pt=3  quantization=Truncate  overflow=Wrap  latency=1  dbl_ovrd=off  pipeline=off  block_type=convert
      settings: block_version=11.4
  convert2 : xbsIndex_r4/Convert  arith_type="Signed  (2's comp)"  n_bits=4  bin_pt=3  quantization=Truncate  overflow=Wrap  latency=1  dbl_ovrd=off  pipeline=off  block_type=convert
      settings: block_version=11.4
  delay : xbsIndex_r4/Delay  en=off  latency=3  dbl_ovrd=off  reg_retiming=off  block_type=delay
      settings: block_version=11.4
  fir_col1 : Subsystem
  fir_col2 : Subsystem
  fir_col3 : Subsystem
  fir_col4 : Subsystem
  imag_sum : Subsystem
      settings: AttributesFormatString=latency 2
  real_sum : Subsystem
      settings: AttributesFormatString=latency 2
  ri_to_c : Subsystem
  shift1 : xbsIndex_r4/Shift  shift_dir=Left  shift_bits=1  en=off  latency=0  precision=Full  arith_type="Signed  (2's comp)"  n_bits=16  bin_pt=14  quantization=Truncate  overflow=Wrap  dbl_ovrd=off  block_type=shift
  shift2 : xbsIndex_r4/Shift  shift_dir=Left  shift_bits=1  en=off  latency=0  precision=Full  arith_type="Signed  (2's comp)"  n_bits=16  bin_pt=14  quantization=Truncate  overflow=Wrap  dbl_ovrd=off  block_type=shift
  sync_out : Outport
  dout : Outport  Port=2
  wires:
  delay/1 -> real_sum/1(sync), imag_sum/1(sync)
  shift2/1 -> convert2/1
  imag_sum/2(dout) -> shift2/1
  shift1/1 -> convert1/1
  real_sum/2(dout) -> shift1/1
  ri_to_c/1(c) -> dout/1
  convert2/1 -> ri_to_c/2(im)
  convert1/1 -> ri_to_c/1(re)
  real_sum/1(sync_out) -> sync_out/1
  fir_col4/3(real_sum) -> real_sum/5(din4)  "xlsub2_real_sum_inports5"
  fir_col3/3(real_sum) -> real_sum/4(din3)  "xlsub2_real_sum_inports4"
  fir_col2/3(real_sum) -> real_sum/3(din2)  "xlsub2_real_sum_inports3"
  fir_col1/3(real_sum) -> real_sum/2(din1)  "xlsub2_real_sum_inports2"
  fir_col4/4(imag_sum) -> imag_sum/5(din4)  "xlsub2_imag_sum_inports5"
  fir_col3/4(imag_sum) -> imag_sum/4(din3)  "xlsub2_imag_sum_inports4"
  fir_col2/4(imag_sum) -> imag_sum/3(din2)  "xlsub2_imag_sum_inports3"
  fir_col1/4(imag_sum) -> imag_sum/2(din1)  "xlsub2_imag_sum_inports2"
  fir_col3/2(imag_out1) -> fir_col4/2(imag1)  "xlsub2_fir_col3_2"
  fir_col3/1(real_out1) -> fir_col4/1(real1)  "xlsub2_fir_col3_1"
  fir_col2/2(imag_out1) -> fir_col3/2(imag1)  "xlsub2_fir_col2_2"
  fir_col2/1(real_out1) -> fir_col3/1(real1)  "xlsub2_fir_col2_1"
  fir_col1/2(imag_out1) -> fir_col2/2(imag1)  "xlsub2_fir_col1_2"
  fir_col1/1(real_out1) -> fir_col2/1(real1)  "xlsub2_fir_col1_1"
  imag1/1 -> fir_col1/2(imag1)
  real1/1 -> fir_col1/1(real1)
  sync_in/1 -> delay/1

== system gbt_library/parallel_fir/f1 ==
  sync_in : Inport
  real1 : Inport  Port=2
  imag1 : Inport  Port=3
  convert1 : xbsIndex_r4/Convert  arith_type="Signed  (2's comp)"  n_bits=4  bin_pt=3  quantization=Truncate  overflow=Wrap  latency=1  dbl_ovrd=off  pipeline=off  block_type=convert
      settings: block_version=11.4
  convert2 : xbsIndex_r4/Convert  arith_type="Signed  (2's comp)"  n_bits=4  bin_pt=3  quantization=Truncate  overflow=Wrap  latency=1  dbl_ovrd=off  pipeline=off  block_type=convert
      settings: block_version=11.4
  delay : xbsIndex_r4/Delay  en=off  latency=3  dbl_ovrd=off  reg_retiming=off  block_type=delay
      settings: block_version=11.4
  fir_col1 : Subsystem
  fir_col2 : Subsystem
  fir_col3 : Subsystem
  fir_col4 : Subsystem
  imag_sum : Subsystem
      settings: AttributesFormatString=latency 2
  real_sum : Subsystem
      settings: AttributesFormatString=latency 2
  ri_to_c : Subsystem
  shift1 : xbsIndex_r4/Shift  shift_dir=Left  shift_bits=1  en=off  latency=0  precision=Full  arith_type="Signed  (2's comp)"  n_bits=16  bin_pt=14  quantization=Truncate  overflow=Wrap  dbl_ovrd=off  block_type=shift
  shift2 : xbsIndex_r4/Shift  shift_dir=Left  shift_bits=1  en=off  latency=0  precision=Full  arith_type="Signed  (2's comp)"  n_bits=16  bin_pt=14  quantization=Truncate  overflow=Wrap  dbl_ovrd=off  block_type=shift
  sync_out : Outport
  dout : Outport  Port=2
  wires:
  delay/1 -> real_sum/1(sync), imag_sum/1(sync)
  shift2/1 -> convert2/1
  imag_sum/2(dout) -> shift2/1
  shift1/1 -> convert1/1
  real_sum/2(dout) -> shift1/1
  ri_to_c/1(c) -> dout/1
  convert2/1 -> ri_to_c/2(im)
  convert1/1 -> ri_to_c/1(re)
  real_sum/1(sync_out) -> sync_out/1
  fir_col4/3(real_sum) -> real_sum/5(din4)  "xlsub2_real_sum_inports5"
  fir_col3/3(real_sum) -> real_sum/4(din3)  "xlsub2_real_sum_inports4"
  fir_col2/3(real_sum) -> real_sum/3(din2)  "xlsub2_real_sum_inports3"
  fir_col1/3(real_sum) -> real_sum/2(din1)  "xlsub2_real_sum_inports2"
  fir_col4/4(imag_sum) -> imag_sum/5(din4)  "xlsub2_imag_sum_inports5"
  fir_col3/4(imag_sum) -> imag_sum/4(din3)  "xlsub2_imag_sum_inports4"
  fir_col2/4(imag_sum) -> imag_sum/3(din2)  "xlsub2_imag_sum_inports3"
  fir_col1/4(imag_sum) -> imag_sum/2(din1)  "xlsub2_imag_sum_inports2"
  fir_col3/2(imag_out1) -> fir_col4/2(imag1)  "xlsub2_fir_col3_2"
  fir_col3/1(real_out1) -> fir_col4/1(real1)  "xlsub2_fir_col3_1"
  fir_col2/2(imag_out1) -> fir_col3/2(imag1)  "xlsub2_fir_col2_2"
  fir_col2/1(real_out1) -> fir_col3/1(real1)  "xlsub2_fir_col2_1"
  fir_col1/2(imag_out1) -> fir_col2/2(imag1)  "xlsub2_fir_col1_2"
  fir_col1/1(real_out1) -> fir_col2/1(real1)  "xlsub2_fir_col1_1"
  imag1/1 -> fir_col1/2(imag1)
  real1/1 -> fir_col1/1(real1)
  sync_in/1 -> delay/1

== system gbt_library/speadizer/Shpacketizer ==
  din_valid : Inport
  din : Inport  Port=2
  sync_reset : Inport  Port=3
  waste_time : Inport  Port=4
  wr_heap : Inport  Port=5
  Counter : xbsIndex_r4/Counter  cnt_type=Free Running  cnt_to=Inf  operation=Up  start_count=0  cnt_by_val=1  arith_type=Unsigned  n_bits=11  bin_pt=0  load_pin=off  rst=on  en=on  explicit_period=on  period=1  dbl_ovrd=off  use_behavioral_HDL=off  implementation=Fabric  use_rpm=off  block_type=counter
  Inverter : xbsIndex_r4/Inverter  en=off  latency=0  dbl_ovrd=off  block_type=inv
  Logical : xbsIndex_r4/Logical  logical_function=AND  inputs=2  en=off  latency=0  precision=Full  arith_type=Unsigned  n_bits=16  bin_pt=0  align_bp=on  dbl_ovrd=off  block_type=logical
  Logical1 : xbsIndex_r4/Logical  logical_function=AND  inputs=2  en=off  latency=0  precision=Full  arith_type=Unsigned  n_bits=16  bin_pt=0  align_bp=on  dbl_ovrd=off  block_type=logical
  data_buffer : xbsIndex_r4/FIFO  depth=2K  percent_nbits=1  rst=off  en=off  use_dcount=off  use_almost_empty=off  almost_empty_thresh=2  use_almost_full=off  almost_full_thresh=14  dbl_ovrd=off  mem_type=Block RAM  explicit_period=off  block_type=fifo
      settings: block_version=10.1.3
  data_counter : xbsIndex_r4/Counter  cnt_type=Free Running  cnt_to=Inf  operation=Up  start_count=0  cnt_by_val=1  arith_type=Unsigned  n_bits=6  bin_pt=0  load_pin=off  rst=on  en=on  explicit_period=on  period=1  dbl_ovrd=off  use_behavioral_HDL=off  implementation=Fabric  use_rpm=off  block_type=counter
  parallel_to_serial_converter : Subsystem  AncestorBlock=casper_library/Flow_Control/parallel_to_serial_converter  mask(parallel_to_serial_converter){pin_width=256, sout_width=64}
      mask prompts: pin_width "Parallel Input Width"; sout_width "Serial Output Width"
      mask help:
      | This block takes as input a parallel bus of specified width.
      | When the load signal 'ld' is asserted, this data is broken into
      | pieces of width specified by the serial output width and
      | stored into different registers chained to form a shift register.
      | If the 'shift' input is subsequently asserted, the shift register
      | returns as output a new piece of data of width sout_width.  This data
      | is the next least significant piece of the original bus.  The converter
      | serializes SMALL ENDIAN.
      |
      | Note that the load operation automatically loads the least significant
      | bits into the register closest to the output, so the first 'shift'
      | assertion changes the data output from bits [sout_width-1:0] to
      | bits [2*sout_width-1:sout_width].
      mask init:
      | parallel_to_serial_converter_init(gcb, ...
      |     'pin_width', pin_width, ...
      |     'sout_width', sout_width);
  shift_counter : xbsIndex_r4/Counter  cnt_type=Free Running  cnt_to=Inf  operation=Up  start_count=0  cnt_by_val=1  arith_type=Unsigned  n_bits=3  bin_pt=0  load_pin=off  rst=on  en=on  explicit_period=on  period=1  dbl_ovrd=off  use_behavioral_HDL=off  implementation=Fabric  use_rpm=off  block_type=counter
  shpacketizer_fsm : xbsIndex_r4/MCode  mfname=shpacketizer_fsm  explicit_period=off  period=1  inputsTable={'boundInpExpr'=>['','','3','','31','','','',''],'inputs'=>['fifo_empty','shift_count','data_per_word','data_count','n_words','sync_reset','waste_count','waste_time','wr_heap']}  outputsTable={'outputs'=>['fifo_re','bram_addr_en','bram_we','serializer_shift','serializer_ld','shift_count_en','shift_count_rst','bram_addr_rst','data_count_en','data_count_rst','done','waste_count_en','waste_count_rst'],'suppressOut'=>['off','off','off','off','off','off','off','off','off','off','off','off','off']}  dbl_ovrd=off  enable_stdout=off  enable_debug=off  suppress_output=on  defparams={'data_per_word',3,'n_words',31}  hide_port_list={}  block_type=mcode
      settings: block_version=11.4
  waste_counter : xbsIndex_r4/Counter  cnt_type=Free Running  cnt_to=Inf  operation=Up  start_count=0  cnt_by_val=1  arith_type=Unsigned  n_bits=5  bin_pt=0  load_pin=off  rst=on  en=on  explicit_period=on  period=1  dbl_ovrd=off  use_behavioral_HDL=off  implementation=Fabric  use_rpm=off  block_type=counter
  data_addr : Outport
  data_sout : Outport  Port=2
  data_valid : Outport  Port=3
  buffer_overflow : Outport  Port=4
  wires:
  waste_counter/1 -> shpacketizer_fsm/5
  sync_reset/1 -> shpacketizer_fsm/4
  data_counter/1 -> shpacketizer_fsm/3
  waste_time/1 -> shpacketizer_fsm/6
  wr_heap/1 -> shpacketizer_fsm/7
  Logical1/1 -> buffer_overflow/1
  data_buffer/4 -> Logical1/2, Inverter/1
  Inverter/1 -> Logical/2
  din_valid/1 -> Logical1/1, Logical/1
  Logical/1 -> data_buffer/2
  data_buffer/1 -> parallel_to_serial_converter/1(pin)
  shpacketizer_fsm/1 -> data_buffer/3
  shpacketizer_fsm/4 -> parallel_to_serial_converter/3(shift)
  shpacketizer_fsm/5 -> parallel_to_serial_converter/2(ld)
  shpacketizer_fsm/3 -> data_valid/1
  din/1 -> data_buffer/1
  parallel_to_serial_converter/1(sout) -> data_sout/1
  shpacketizer_fsm/6 -> shift_counter/2
  shift_counter/1 -> shpacketizer_fsm/2
  shpacketizer_fsm/7 -> shift_counter/1
  data_buffer/2 -> shpacketizer_fsm/1
  Counter/1 -> data_addr/1
  shpacketizer_fsm/2 -> Counter/2
  shpacketizer_fsm/8 -> Counter/1
  shpacketizer_fsm/9 -> data_counter/2
  shpacketizer_fsm/10 -> data_counter/1
  shpacketizer_fsm/12 -> waste_counter/2
  shpacketizer_fsm/13 -> waste_counter/1
